simulink model "StereoImageRectificationHDL2020a"  (R2020a)
settings: Solver=FixedStepDiscrete  StartTime=0.0  StopTime=totalPixels*totalLines  FixedStep=1  RelTol=1e-3
InitFcn:
  | load('stereoParams.mat');
  | img = imread(get_param('StereoImageRectificationHDL2020a/LeftInputImage','FileName'));
  | dimOut=size(img);
  | [imgRowSize, imgColSize] = size(img);
  | run('ComputeRectificationParams.m');
values from neighbouring files (symbols this model uses):
  displacement = maxDev+firstRow    [ComputeRectificationParams.m]
  distCoeffsL = [this.CameraParameters1.RadialDistortion, this.CameraParameters1.TangentialDistortion]    [ComputeRectificationParams.m]
  distCoeffsR = [this.CameraParameters2.RadialDistortion, this.CameraParameters2.TangentialDistortion]    [ComputeRectificationParams.m]
  offset = displacement+50    [ComputeRectificationParams.m]
  recleftfx = 1/intrinsicL(1,1)    [ComputeRectificationParams.m]
  recleftfy = 1/intrinsicL(2,2)    [ComputeRectificationParams.m]
  recrightfx = 1/intrinsicR(1,1)    [ComputeRectificationParams.m]
  recrightfy = 1/intrinsicR(2,2)    [ComputeRectificationParams.m]
  totalLines = R + 100    (= 580)    [setup.m]
  totalPixels = C + frontPorch    (= 802)    [setup.m]
undefined symbols (not defined in the file or in its folder): gray, imgColSize, imgRowSize, intrinsicL, intrinsicR, leftH, rightH, XBounds, YBounds
libraries: simulink x62, hdlsllib x30, visionhdlio x4, visionsources x2, visionhdlutilities x1
(part 3 of 3)

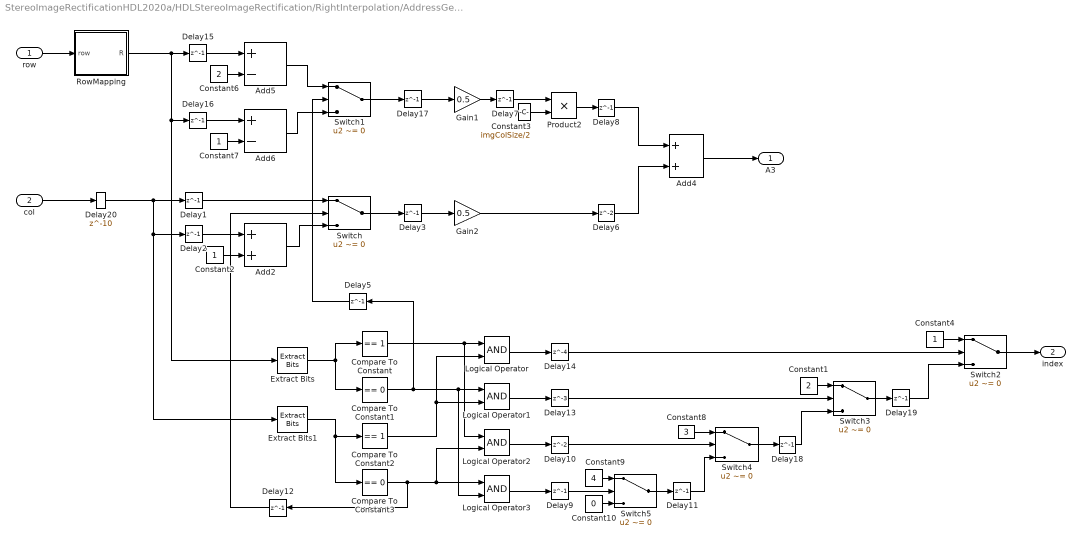
== system StereoImageRectificationHDL2020a/HDLStereoImageRectification/RightInterpolation/AddressGeneration/AddressCalculation/Pix3Add ==
  row : Inport
  col : Inport  Port=2
  Add2 : Sum  OutDataTypeStr=Inherit: Same as first input
  Add4 : Sum  OutDataTypeStr=Inherit: Same as first input
  Add5 : Sum  Inputs=+-  OutDataTypeStr=Inherit: Same as first input
  Add6 : Sum  Inputs=+-  OutDataTypeStr=Inherit: Same as first input
  Compare To Constant : simulink/Logic and Bit Operations/Compare To Constant  relop===  const=1  OutDataTypeStr=boolean
  Compare To Constant1 : simulink/Logic and Bit Operations/Compare To Constant  relop===  const=0  OutDataTypeStr=boolean
  Compare To Constant2 : simulink/Logic and Bit Operations/Compare To Constant  relop===  const=1  OutDataTypeStr=boolean
  Compare To Constant3 : simulink/Logic and Bit Operations/Compare To Constant  relop===  const=0  OutDataTypeStr=boolean
  Constant1 : Constant  Value=2  OutDataTypeStr=uint8  SampleTime=-1
  Constant10 : Constant  Value=0  OutDataTypeStr=uint8  SampleTime=-1
  Constant2 : Constant  OutDataTypeStr=Inherit: Inherit via back propagation  SampleTime=-1
  Constant3 : Constant  Value=imgColSize/2  OutDataTypeStr=uint32  SampleTime=-1
  Constant4 : Constant  OutDataTypeStr=uint8  SampleTime=-1
  Constant6 : Constant  Value=2  OutDataTypeStr=Inherit: Inherit via back propagation  SampleTime=-1
  Constant7 : Constant  OutDataTypeStr=Inherit: Inherit via back propagation  SampleTime=-1
  Constant8 : Constant  Value=3  OutDataTypeStr=uint8  SampleTime=-1
  Constant9 : Constant  Value=4  OutDataTypeStr=uint8  SampleTime=-1
  Delay{1..3,5,7..9,11..12,15..19} (14 alike) : Delay  DelayLength=1
  Delay10 : Delay
  Delay13 : Delay  DelayLength=3
  Delay14 : Delay  DelayLength=4
  Delay20 : Delay  DelayLength=10
  Delay6 : Delay
  Extract Bits : simulink/Logic and Bit Operations/Extract Bits  bitsToExtract=Range ending with least significant bit  numBits=1  bitIdxRange=[0 7]  outScalingMode=Preserve fixed-point scaling
  Extract Bits1 : simulink/Logic and Bit Operations/Extract Bits  bitsToExtract=Range ending with least significant bit  numBits=1  bitIdxRange=[0 7]  outScalingMode=Preserve fixed-point scaling
  Gain1 : Gain  Gain=0.5  OutDataTypeStr=Inherit: Inherit via back propagation
  Gain2 : Gain  Gain=0.5  OutDataTypeStr=Inherit: Inherit via back propagation
  Logical Operator{,1..3} (4 alike) : Logic  AllPortsSameDT=off  OutDataTypeStr=boolean
  Product2 : Product  OutDataTypeStr=Inherit: Inherit via back propagation
  RowMapping : Subsystem
  Switch{,1..5} (6 alike) : Switch  Criteria=u2 ~= 0
  A3 : Outport
  index : Outport  Port=2
  wires:
  Gain2/1 -> Delay6/1
  Switch/1 -> Delay3/1
  Delay3/1 -> Gain2/1
  Delay2/1 -> Add2/1
  Constant2/1 -> Add2/2
  Delay1/1 -> Switch/1
  Add2/1 -> Switch/3
  Delay5/1 -> Switch1/2
  Delay17/1 -> Gain1/1
  Switch1/1 -> Delay17/1
  Add6/1 -> Switch1/3
  Add5/1 -> Switch1/1
  Constant7/1 -> Add6/2
  Delay16/1 -> Add6/1
  Delay15/1 -> Add5/1
  Constant6/1 -> Add5/2
  Gain1/1 -> Delay7/1
  Constant3/1 -> Product2/2
  Delay7/1 -> Product2/1
  Product2/1 -> Delay8/1
  Delay8/1 -> Add4/1
  Delay6/1 -> Add4/2
  Add4/1 -> A3/1
  Extract Bits/1 -> Compare To Constant/1, Compare To Constant1/1
  Extract Bits1/1 -> Compare To Constant3/1, Compare To Constant2/1
  Compare To Constant/1 -> Logical Operator2/1, Logical Operator/1
  Compare To Constant2/1 -> Logical Operator1/2, Logical Operator/2
  Compare To Constant1/1 -> Delay5/1, Logical Operator3/2, Logical Operator1/1
  Switch2/1 -> index/1
  Compare To Constant3/1 -> Logical Operator3/1, Logical Operator2/2, Delay12/1
  Delay12/1 -> Switch/2
  col/1 -> Delay20/1
  Delay14/1 -> Switch2/2
  Delay11/1 -> Switch4/3
  Delay19/1 -> Switch2/3
  Switch5/1 -> Delay11/1
  Delay9/1 -> Switch5/2
  Constant1/1 -> Switch3/1
  Constant10/1 -> Switch5/3
  Delay13/1 -> Switch3/2
  Constant4/1 -> Switch2/1
  Switch4/1 -> Delay18/1
  Delay10/1 -> Switch4/2
  Constant9/1 -> Switch5/1
  Switch3/1 -> Delay19/1
  Constant8/1 -> Switch4/1
  Delay18/1 -> Switch3/3
  Logical Operator3/1 -> Delay9/1
  Logical Operator2/1 -> Delay10/1
  Logical Operator1/1 -> Delay13/1
  Logical Operator/1 -> Delay14/1
  RowMapping/1(R) -> Delay15/1, Extract Bits/1, Delay16/1
  row/1 -> RowMapping/1(row)
  Delay20/1 -> Delay1/1, Extract Bits1/1, Delay2/1

== system StereoImageRectificationHDL2020a/HDLStereoImageRectification/RightInterpolation/AddressGeneration/AddressCalculation/Pix4Add ==
  A3 : Inport
  Index : Inport  Port=2
  Add : Sum  OutDataTypeStr=Inherit: Inherit via back propagation
  Add2 : Sum  OutDataTypeStr=Inherit: Inherit via back propagation
  Add3 : Sum  Inputs=+-  OutDataTypeStr=Inherit: Inherit via back propagation
  Compare To Constant : simulink/Logic and Bit Operations/Compare To Constant  relop===  const=1  OutDataTypeStr=boolean
  Compare To Constant1 : simulink/Logic and Bit Operations/Compare To Constant  relop===  const=2  OutDataTypeStr=boolean
  Constant : Constant  OutDataTypeStr=Inherit: Inherit via back propagation  SampleTime=-1
  Constant1 : Constant  Value=2  OutDataTypeStr=Inherit: Inherit via back propagation  SampleTime=-1
  Constant2 : Constant  Value=2  OutDataTypeStr=Inherit: Inherit via back propagation  SampleTime=-1
  Delay{,1..12} (13 alike) : Delay  DelayLength=1
  Logical Operator : Logic  Operator=OR  AllPortsSameDT=off  OutDataTypeStr=boolean
  Switch : Switch  Criteria=u2 ~= 0
  Switch1 : Switch  Criteria=u2 ~= 0
  A4 : Outport
  index : Outport  Port=2
  wires:
  Compare To Constant/1 -> Delay2/1
  Compare To Constant1/1 -> Delay3/1
  Logical Operator/1 -> Delay6/1
  A3/1 -> Delay1/1
  Switch/1 -> A4/1
  Constant/1 -> Add/2
  Add/1 -> Delay8/1
  Add2/1 -> Delay11/1
  Constant1/1 -> Add2/2
  Switch1/1 -> index/1
  Constant2/1 -> Add3/2
  Index/1 -> Delay/1
  Add3/1 -> Delay12/1
  Delay/1 -> Compare To Constant/1, Compare To Constant1/1, Delay9/1, Delay10/1
  Delay1/1 -> Delay5/1, Delay4/1
  Delay2/1 -> Logical Operator/1
  Delay3/1 -> Logical Operator/2
  Delay4/1 -> Delay7/1
  Delay5/1 -> Add/1
  Delay6/1 -> Switch1/2, Switch/2
  Delay7/1 -> Switch/1
  Delay8/1 -> Switch/3
  Delay9/1 -> Add2/1
  Delay10/1 -> Add3/1
  Delay11/1 -> Switch1/1
  Delay12/1 -> Switch1/3

== system StereoImageRectificationHDL2020a/HDLStereoImageRectification/LeftInterpolation/AddressGeneration/AddressCalculation/Pix1Add/Row mapping ==
  row : Inport
  Add1 : Sum  Inputs=+-  OutDataTypeStr=Inherit: Same as first input
  Add4 : Sum  Inputs=+-  OutDataTypeStr=Inherit: Same as first input
  Constant : Constant  Value=1/offset  OutDataTypeStr=fixdt(0,16,22)  SampleTime=-1
  Constant4 : Constant  OutDataTypeStr=Inherit: Inherit via back propagation  SampleTime=-1
  Constant5 : Constant  Value=offset  OutDataTypeStr=uint8  SampleTime=-1
  Constant6 : Constant  Value=2  OutDataTypeStr=Inherit: Inherit via back propagation  SampleTime=-1
  Data Type Conversion1 : DataTypeConversion  OutDataTypeStr=uint8
  Delay : Delay  DelayLength=1
  Delay1 : Delay  DelayLength=1
  Delay{2..7} (6 alike) : Delay
  Delay8 : Delay  DelayLength=9
  Delay9 : Delay  DelayLength=1
  Product1 : Product
  Product2 : Product  OutDataTypeStr=uint8
  Switch1 : Switch  Threshold=2  OutDataTypeStr=Inherit: Inherit via back propagation
  R : Outport
  wires:
  row/1 -> Switch1/1, Delay8/1, Switch1/2
  Product1/1 -> Delay7/1
  Constant6/1 -> Switch1/3
  Switch1/1 -> Delay/1
  Constant/1 -> Delay3/1
  Product2/1 -> Delay4/1
  Add1/1 -> Delay2/1
  Constant5/1 -> Delay6/1
  Data Type Conversion1/1 -> Delay5/1
  Add4/1 -> Delay9/1
  Constant4/1 -> Delay1/1
  Delay/1 -> Add1/1
  Delay1/1 -> Add1/2
  Delay2/1 -> Product2/1
  Delay3/1 -> Product2/2
  Delay4/1 -> Data Type Conversion1/1
  Delay5/1 -> Product1/1
  Delay6/1 -> Product1/2
  Delay7/1 -> Add4/2
  Delay8/1 -> Add4/1
  Delay9/1 -> R/1

== system StereoImageRectificationHDL2020a/HDLStereoImageRectification/LeftInterpolation/AddressGeneration/AddressCalculation/Pix3Add/RowMapping ==
  row : Inport
  Add1 : Sum  Inputs=+-  OutDataTypeStr=Inherit: Same as first input
  Add4 : Sum  Inputs=+-  OutDataTypeStr=Inherit: Same as first input
  Constant : Constant  Value=1/offset  OutDataTypeStr=fixdt(0,16,22)  SampleTime=-1
  Constant4 : Constant  OutDataTypeStr=Inherit: Inherit via back propagation  SampleTime=-1
  Constant5 : Constant  Value=offset  OutDataTypeStr=uint8  SampleTime=-1
  Constant6 : Constant  Value=2  OutDataTypeStr=Inherit: Inherit via back propagation  SampleTime=-1
  Data Type Conversion1 : DataTypeConversion  OutDataTypeStr=uint8
  Delay : Delay  DelayLength=1
  Delay1 : Delay  DelayLength=1
  Delay{2..7} (6 alike) : Delay
  Delay8 : Delay  DelayLength=9
  Delay9 : Delay  DelayLength=1
  Product1 : Product
  Product2 : Product  OutDataTypeStr=uint8
  Switch1 : Switch  Threshold=2  OutDataTypeStr=Inherit: Inherit via back propagation
  R : Outport
  wires:
  row/1 -> Switch1/1, Delay8/1, Switch1/2
  Product1/1 -> Delay7/1
  Constant6/1 -> Switch1/3
  Switch1/1 -> Delay/1
  Constant/1 -> Delay3/1
  Product2/1 -> Delay4/1
  Add1/1 -> Delay2/1
  Constant5/1 -> Delay6/1
  Data Type Conversion1/1 -> Delay5/1
  Add4/1 -> Delay9/1
  Constant4/1 -> Delay1/1
  Delay/1 -> Add1/1
  Delay1/1 -> Add1/2
  Delay2/1 -> Product2/1
  Delay3/1 -> Product2/2
  Delay4/1 -> Data Type Conversion1/1
  Delay5/1 -> Product1/1
  Delay6/1 -> Product1/2
  Delay7/1 -> Add4/2
  Delay8/1 -> Add4/1
  Delay9/1 -> R/1

== system StereoImageRectificationHDL2020a/HDLStereoImageRectification/RightInterpolation/AddressGeneration/AddressCalculation/Pix1Add/RowMapping ==
  row : Inport
  Add1 : Sum  Inputs=+-  OutDataTypeStr=Inherit: Same as first input
  Add4 : Sum  Inputs=+-  OutDataTypeStr=Inherit: Same as first input
  Constant : Constant  Value=1/offset  OutDataTypeStr=fixdt(0,16,22)  SampleTime=-1
  Constant4 : Constant  OutDataTypeStr=Inherit: Inherit via back propagation  SampleTime=-1
  Constant5 : Constant  Value=offset  OutDataTypeStr=uint8  SampleTime=-1
  Constant6 : Constant  Value=2  OutDataTypeStr=Inherit: Inherit via back propagation  SampleTime=-1
  Data Type Conversion1 : DataTypeConversion  OutDataTypeStr=uint8
  Delay : Delay  DelayLength=1
  Delay1 : Delay  DelayLength=1
  Delay{2..7} (6 alike) : Delay
  Delay8 : Delay  DelayLength=9
  Delay9 : Delay  DelayLength=1
  Product1 : Product
  Product2 : Product  OutDataTypeStr=uint8
  Switch1 : Switch  Threshold=2  OutDataTypeStr=Inherit: Inherit via back propagation
  R : Outport
  wires:
  row/1 -> Switch1/1, Delay8/1, Switch1/2
  Product1/1 -> Delay7/1
  Constant6/1 -> Switch1/3
  Switch1/1 -> Delay/1
  Constant/1 -> Delay3/1
  Product2/1 -> Delay4/1
  Add1/1 -> Delay2/1
  Constant5/1 -> Delay6/1
  Data Type Conversion1/1 -> Delay5/1
  Add4/1 -> Delay9/1
  Constant4/1 -> Delay1/1
  Delay/1 -> Add1/1
  Delay1/1 -> Add1/2
  Delay2/1 -> Product2/1
  Delay3/1 -> Product2/2
  Delay4/1 -> Data Type Conversion1/1
  Delay5/1 -> Product1/1
  Delay6/1 -> Product1/2
  Delay7/1 -> Add4/2
  Delay8/1 -> Add4/1
  Delay9/1 -> R/1

== system StereoImageRectificationHDL2020a/HDLStereoImageRectification/RightInterpolation/AddressGeneration/AddressCalculation/Pix3Add/RowMapping ==
  row : Inport
  Add1 : Sum  Inputs=+-  OutDataTypeStr=Inherit: Same as first input
  Add4 : Sum  Inputs=+-  OutDataTypeStr=Inherit: Same as first input
  Constant : Constant  Value=1/offset  OutDataTypeStr=fixdt(0,16,22)  SampleTime=-1
  Constant4 : Constant  OutDataTypeStr=Inherit: Inherit via back propagation  SampleTime=-1
  Constant5 : Constant  Value=offset  OutDataTypeStr=uint8  SampleTime=-1
  Constant6 : Constant  Value=2  OutDataTypeStr=Inherit: Inherit via back propagation  SampleTime=-1
  Data Type Conversion1 : DataTypeConversion  OutDataTypeStr=uint8
  Delay : Delay  DelayLength=1
  Delay1 : Delay  DelayLength=1
  Delay{2..7} (6 alike) : Delay
  Delay8 : Delay  DelayLength=9
  Delay9 : Delay  DelayLength=1
  Product1 : Product
  Product2 : Product  OutDataTypeStr=uint8
  Switch1 : Switch  Threshold=2  OutDataTypeStr=Inherit: Inherit via back propagation
  R : Outport
  wires:
  row/1 -> Switch1/1, Delay8/1, Switch1/2
  Product1/1 -> Delay7/1
  Constant6/1 -> Switch1/3
  Switch1/1 -> Delay/1
  Constant/1 -> Delay3/1
  Product2/1 -> Delay4/1
  Add1/1 -> Delay2/1
  Constant5/1 -> Delay6/1
  Data Type Conversion1/1 -> Delay5/1
  Add4/1 -> Delay9/1
  Constant4/1 -> Delay1/1
  Delay/1 -> Add1/1
  Delay1/1 -> Add1/2
  Delay2/1 -> Product2/1
  Delay3/1 -> Product2/2
  Delay4/1 -> Data Type Conversion1/1
  Delay5/1 -> Product1/1
  Delay6/1 -> Product1/2
  Delay7/1 -> Add4/2
  Delay8/1 -> Add4/1
  Delay9/1 -> R/1

== matlab function StereoImageRectificationHDL2020a/HDLStereoImageRectification/LeftInterpolation/AddressGeneration/AddressCalculation/IndexChangeForMemoryAccess ==
  data: add input; Add_Re output; index input; Index_Re output

function [Add_Re, Index_Re]= fcn(add, index)
%#codegen
z=add;
leftInd=index;
if index(1)==1
    z(1)=add(1);
    leftInd(1)=uint8(1);
elseif index(2)==1
    z(1)=add(2);
    leftInd(1)=uint8(2);
elseif index(3)==1
    z(1)=add(3);
    leftInd(1)=uint8(3);
elseif index(4)==1
    z(1)=add(4);
    leftInd(1)=uint8(4);
end

if index(1)==2
    z(2)=add(1);
    leftInd(2)=uint8(1);
elseif index(2)==2
    z(2)=add(2);
    leftInd(2)=uint8(2);
elseif index(3)==2
    z(2)=add(3);
    leftInd(2)=uint8(3);
elseif index(4)==2
    z(2)=add(4);
    leftInd(2)=uint8(4);
end    

if index(1)==3
    z(3)=add(1);
    leftInd(3)=uint8(1);
elseif index(2)==3
    z(3)=add(2);
    leftInd(3)=uint8(2);
elseif index(3)==3
    z(3)=add(3);
    leftInd(3)=uint8(3);
elseif index(4)==3
    z(3)=add(4);
    leftInd(3)=uint8(4);
end    

if index(1)==4
    z(4)=add(1);
    leftInd(4)=uint8(1);
elseif index(2)==4
    z(4)=add(2);
    leftInd(4)=uint8(2);   
elseif index(3)==4
    z(4)=add(3);
    leftInd(4)=uint8(3);
elseif index(4)==4
    z(4)=add(4);
    leftInd(4)=uint8(4);
end  
Add_Re=z;
Index_Re=leftInd;

== matlab function StereoImageRectificationHDL2020a/HDLStereoImageRectification/LeftInterpolation/BilinearInterpolation/IndexChangeForInterpolation ==
  data: pixelValue input; pixOut output; index input
function pixOut = fcn(pixelValue, index)
%#codegen
z=pixelValue;
if index(1)==1
    z(1)=pixelValue(1);
elseif index(2)==1
    z(1)=pixelValue(2);
elseif index(3)==1
    z(1)=pixelValue(3);
elseif index(4)==1
    z(1)=pixelValue(4);
end

if index(1)==2
    z(2)=pixelValue(1);
elseif index(2)==2
    z(2)=pixelValue(2);
elseif index(3)==2
    z(2)=pixelValue(3);
elseif index(4)==2
    z(2)=pixelValue(4);
end    

if index(1)==3
    z(3)=pixelValue(1);
elseif index(2)==3
    z(3)=pixelValue(2);
elseif index(3)==3
    z(3)=pixelValue(3);
elseif index(4)==3
    z(3)=pixelValue(4);
end    

if index(1)==4
    z(4)=pixelValue(1);
elseif index(2)==4
    z(4)=pixelValue(2);
elseif index(3)==4
    z(4)=pixelValue(3);
elseif index(4)==4
    z(4)=pixelValue(4);
end  
pixOut=z';

== matlab function StereoImageRectificationHDL2020a/HDLStereoImageRectification/RightInterpolation/BilinearInterpolation/IndexChangeForInterpolation ==
  data: pixelValue input; pixOut output; index input
function pixOut = fcn(pixelValue, index)
%#codegen
z=pixelValue;
if index(1)==1
    z(1)=pixelValue(1);
elseif index(2)==1
    z(1)=pixelValue(2);
elseif index(3)==1
    z(1)=pixelValue(3);
elseif index(4)==1
    z(1)=pixelValue(4);
end

if index(1)==2
    z(2)=pixelValue(1);
elseif index(2)==2
    z(2)=pixelValue(2);
elseif index(3)==2
    z(2)=pixelValue(3);
elseif index(4)==2
    z(2)=pixelValue(4);
end    

if index(1)==3
    z(3)=pixelValue(1);
elseif index(2)==3
    z(3)=pixelValue(2);
elseif index(3)==3
    z(3)=pixelValue(3);
elseif index(4)==3
    z(3)=pixelValue(4);
end    

if index(1)==4
    z(4)=pixelValue(1);
elseif index(2)==4
    z(4)=pixelValue(2);
elseif index(3)==4
    z(4)=pixelValue(3);
elseif index(4)==4
    z(4)=pixelValue(4);
end  
pixOut=z';

== matlab function StereoImageRectificationHDL2020a/HDLStereoImageRectification/RightInterpolation/AddressGeneration/AddressCalculation/IndexChangeForMemoryAccess ==
  data: add input; Add_Re output; index input; Index_Re output

function [Add_Re, Index_Re]= fcn(add, index)
%#codegen
z=add;
leftInd=index;
if index(1)==1
    z(1)=add(1);
    leftInd(1)=uint8(1);
elseif index(2)==1
    z(1)=add(2);
    leftInd(1)=uint8(2);
elseif index(3)==1
    z(1)=add(3);
    leftInd(1)=uint8(3);
elseif index(4)==1
    z(1)=add(4);
    leftInd(1)=uint8(4);
end

if index(1)==2
    z(2)=add(1);
    leftInd(2)=uint8(1);
elseif index(2)==2
    z(2)=add(2);
    leftInd(2)=uint8(2);
elseif index(3)==2
    z(2)=add(3);
    leftInd(2)=uint8(3);
elseif index(4)==2
    z(2)=add(4);
    leftInd(2)=uint8(4);
end    

if index(1)==3
    z(3)=add(1);
    leftInd(3)=uint8(1);
elseif index(2)==3
    z(3)=add(2);
    leftInd(3)=uint8(2);
elseif index(3)==3
    z(3)=add(3);
    leftInd(3)=uint8(3);
elseif index(4)==3
    z(3)=add(4);
    leftInd(3)=uint8(4);
end    

if index(1)==4
    z(4)=add(1);
    leftInd(4)=uint8(1);
elseif index(2)==4
    z(4)=add(2);
    leftInd(4)=uint8(2);   
elseif index(3)==4
    z(4)=add(3);
    leftInd(4)=uint8(3);
elseif index(4)==4
    z(4)=add(4);
    leftInd(4)=uint8(4);
end  
Add_Re=z;
Index_Re=leftInd;
